simulink model "simulink_model"  (R2016a)
settings: Solver=ode2  StartTime=0.0  StopTime=1000  FixedStep=1  RelTol=1e-3
settings Model: Creator=Harsh  LastModifiedBy=Harsh

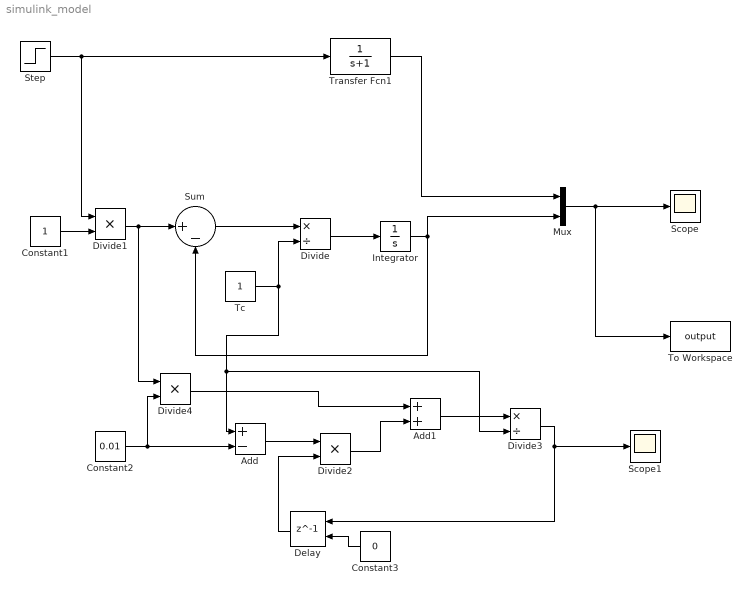
== system simulink_model ==
  Add : Sum  Inputs=+-
  Add1 : Sum
  Constant1 : Constant
  Constant2 : Constant  Value=0.01
  Constant3 : Constant  Value=0
  Delay : Delay  DelayLength=1  InitialConditionSource=Input port
      settings: InputPortMap=u0,p4
  Divide : Product  Inputs=*/
  Divide1 : Product  Inputs=**
  Divide2 : Product  Inputs=**
  Divide3 : Product  Inputs=*/
  Divide4 : Product  Inputs=**
  Integrator : Integrator
  Mux : Mux  Inputs=2
  Scope : Scope
  Scope1 : Scope
  Step : Step  SampleTime=0
  Sum : Sum  Inputs=|+-
  Tc : Constant
  To Workspace : ToWorkspace  VariableName=output  SampleTime=-1
  Transfer Fcn1 : TransferFcn  Denominator=[1 1]
  wires:
  Transfer Fcn1/1 -> Mux/1
  Step/1 -> Divide1/1, Transfer Fcn1/1
  Sum/1 -> Divide/1
  Divide/1 -> Integrator/1
  Divide1/1 -> Divide4/1, Sum/1
  Constant1/1 -> Divide1/2
  Integrator/1 -> Sum/2, Mux/2
  Mux/1 -> To Workspace/1, Scope/1
  Constant2/1 -> Divide4/2, Add/2
  Add/1 -> Divide2/1
  Delay/1 -> Divide2/2
  Divide2/1 -> Add1/2
  Add1/1 -> Divide3/1
  Tc/1 -> Divide3/2, Add/1, Divide/2
  Divide3/1 -> Scope1/1, Delay/1
  Constant3/1 -> Delay/2
  Divide4/1 -> Add1/1
